simulink model "MPCSimulationSlowest"  (Simulink 7.9)
settings: Solver=ode45  StartTime=0.0  StopTime=10  RelTol=1e-3
values from neighbouring files (symbols this model uses):
  A = Plant.A    [MPCController.m]    (also in SlowMPCController.m; SlowestMPCController.m; setupsimulation.m)
  B = Plant.B    [MPCController.m]    (also in SlowMPCController.m; SlowestMPCController.m; setupsimulation.m)
  C = Plant.C    [MPCController.m]    (also in SlowMPCController.m; SlowestMPCController.m; setupsimulation.m)
  Ts = 0.1    [MPCController.m]    (also in SlowMPCController.m; SlowestMPCController.m; setupsimulation.m)
  x0 = [1;1]    [setupsimulation.m]
undefined symbols (not defined in the file or in its folder): SlowestMPCController
settings Model: Creator=johanl  LastModifiedBy=johanl

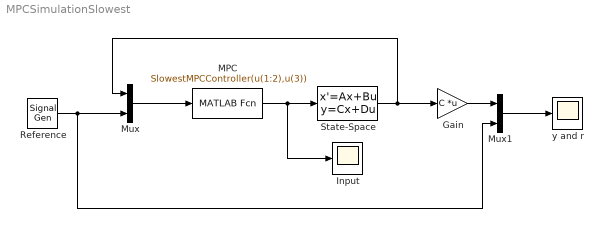
== system MPCSimulationSlowest ==
  Gain : Gain  Gain=C  Multiplication=Matrix(K*u)
  Input : Scope
  MPC : MATLABFcn  MATLABFcn=SlowestMPCController(u(1:2),u(3))  SampleTime=Ts
  Mux : Mux  Inputs=2
  Mux1 : Mux  Inputs=2
  Reference : SignalGenerator  WaveForm=square  Frequency=0.2
  State-Space : StateSpace  A=A  B=B  C=eye(2)  D=zeros(2,1)  X0=x0
  y and r : Scope
  wires:
  State-Space/1 -> Mux/1, Gain/1
  MPC/1 -> State-Space/1, Input/1
  Mux/1 -> MPC/1
  Reference/1 -> Mux/2, Mux1/2
  Gain/1 -> Mux1/1
  Mux1/1 -> y and r/1
